simulink library "Navigation_Lib"  (Simulink 7.5)
settings: Solver=ode45  SolverMode=SingleTasking  StartTime=0.0  StopTime=10.0  RelTol=1e-3
values from neighbouring files (symbols this model uses):
  Env =     [UAV_modelconfig.mat]
undefined symbols (not defined in the file or in its folder): Earth, WGS84
libraries: simulink x2, aerolibtransform2 x1
settings Model: Creator=Paul Freeman  LastModifiedBy=ultrastick

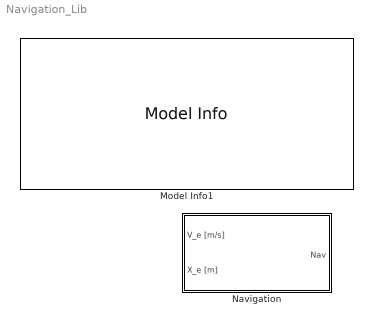
== system Navigation_Lib ==
  Model Info1 : simulink/Model-Wide Utilities/Model Info  SystemSampleTime=-1  InitialBlockCM=None  BlockCM=None  Frame=on  DisplayStringWithTags=|  HorizontalTextAlignment=Left  LeftAlignmentValue=0.02  SourceBlockDiagram=Navigation_Lib  TagMaxNumber=20
      | MODEL INFORMATION
      | Navigation Library
      | 
      | University of Minnesota
      | Aerospace Engineering and Mechanics
      | Copyright 2011 Regents of the University of Minnesota. All rights reserved.
      | 
      | == SVN Info ==
      | %<ModelVersion>
      | Last modified by %<LastModifiedBy> on %<LastModificationDate>
  Navigation : Subsystem  Description=|
      | This model produces the followng navigation data for the UAV flight:
      |                                                                     
      | * Geodetic Latitude                                                 
      | * Geodetic Longitude                                                
      | * Geodetic Altitude                                                 
      | * Altitude above Mean Sea Level                                     
      | * Gravitational acceleration vector

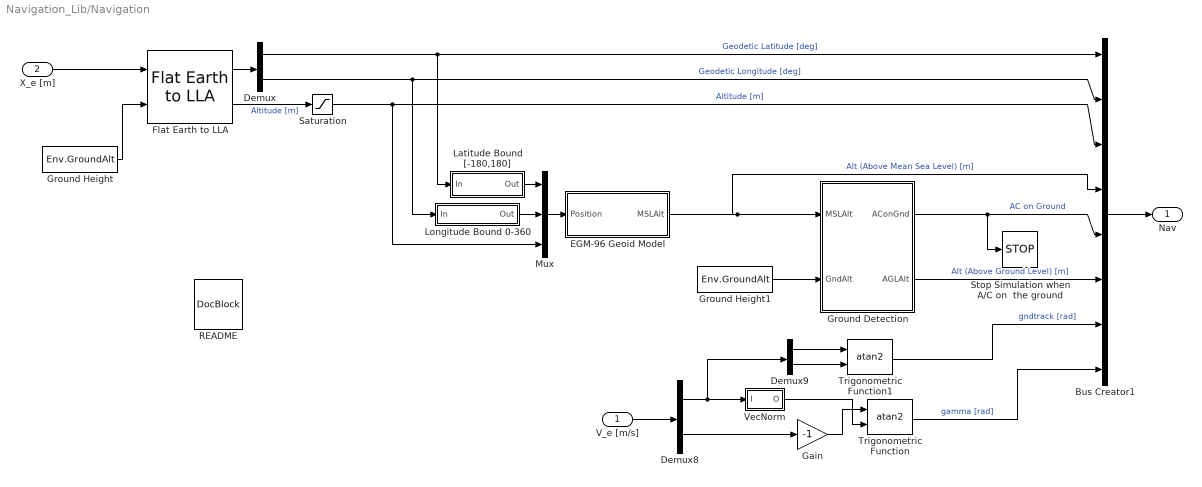
== system Navigation_Lib/Navigation ==
  V_e [m/s] : Inport  OutDataType=sfix(16)  OutScaling=2^0
  X_e [m] : Inport  Port=2  OutDataType=sfix(16)  OutScaling=2^0
  Bus Creator1 : BusCreator  Inputs=8
  Demux : Demux  Outputs=2
  Demux8 : Demux  Outputs=[2 1]
  Demux9 : Demux  Outputs=2
  EGM-96 Geoid Model : Subsystem  mask(EGM-96 geoid undulation model){}
      mask help: Computes the MSL (mean sea level) altitude as a function of position.
      mask init:
      | load('egm96');
      mask Help:
      | The block computes the mean-sea-level altitude relative to the WGS-84 geoid.
      | <P><B>Inputs:</B>
      | <LI>Position = the 3x1 vector of aircraft location [Latitude Longitude Altitude], in [rad rad m]</LI>
      | </P>
      | <P><B>Output:</B>
      | <LI>MSLAlt = the mean-sea-level altitude, in m</LI>
      | </P>
  Flat Earth to LLA : aerolibtransform2/Flat Earth to LLA  SystemSampleTime=-1  units=Metric (MKS)  ptype=Earth (WGS84)  F=1/298.257223563  R=6378137  LL0=TrimCondition.LLIni  psi=0
  Gain : Gain  Gain=-1  ParameterDataType=fixdt(1, 16)  ParameterScaling=2^0  OutDataType=fixdt(1, 16)  OutScaling=2^0
  Ground Detection : Subsystem
      mask Type: Ground detection
      mask Description: Computes altitude above ground and sets a flag if AGL is negative.
      mask Help:
      | The block computes the altitude above ground (AGL) and sets a flag if the AGL is negative (used for ground contact detection).
      | <P><B>Inputs:</B>
      | <LI>MSLAlt = the altitude measured from mean-sea-level, in meters</LI>
      | <LI>GndAlt = the altitude of the terrain (above MSL) at current location, in meters</LI>
      | </P>
      | <P><B>Output:</B>
      | <LI>AConGnd = the aircraft-on-ground flag (0 if aircraft above ground, 1 if aircraft on the ground)</LI>
      | <LI>AGLAlt = the altitude of the aircraft above ground</LI>
      | </P>
  Ground Height : Constant  Value=Env.GroundAlt  OutDataType=sfix(16)  OutScaling=2^0
  Ground Height1 : Constant  Value=Env.GroundAlt  OutDataType=sfix(16)  OutScaling=2^0
  Latitude Bound [-180,180] : Subsystem
  Longitude Bound 0-360 : Subsystem
      mask Type: Longitude bound
      mask Description: Bounds the longitude to [0, 2pi]. When 0 bound is exceeded the longitude wraps back to 2pi; when the 2pi bound is exceeded the longitude wraps back to 0.
  Mux : Mux  Inputs=3
  README : simulink/Model-Wide Utilities/DocBlock  SystemSampleTime=-1  DocumentType=Text
      content=|
      | Navigation
      |
      | This block is library link that contains the navigational model and
      | equations. Included are equations relating the flat Earth position to
      | latitude/longitude, a simplified 2D table lookup version of the EGM-96
      | Geoid model for computation of MSL/AGL altitudes, and computation of
      | flight path and ground track angles.
  Saturation : Saturate  UpperLimit=Inf  LowerLimit=0  OutDataType=fixdt(1, 16)  OutScaling=2^0
  Stop Simulation when A/C on  the ground : Stop
  Trigonometric Function : Trigonometry  Operator=atan2
  Trigonometric Function1 : Trigonometry  Operator=atan2
  VecNorm : Subsystem
  Nav : Outport  OutDataType=sfix(16)  OutScaling=2^0
  wires:
  Flat Earth to LLA/1 -> Demux/1
  Flat Earth to LLA/2 -> Saturation/1  "Altitude [m]"
  Demux/1 -> Bus Creator1/1, Latitude Bound [-180,180]/1(In)  "Geodetic Latitude [deg]"
  Demux/2 -> Bus Creator1/2, Longitude Bound 0-360/1(In)  "Geodetic Longitude [deg]"
  X_e [m]/1 -> Flat Earth to LLA/1
  Ground Height/1 -> Flat Earth to LLA/2
  Bus Creator1/1 -> Nav/1
  EGM-96 Geoid Model/1(MSLAlt) -> Ground Detection/1(MSLAlt), Bus Creator1/4  "Alt (Above Mean Sea Level) [m]"
  Ground Height1/1 -> Ground Detection/2(GndAlt)
  Ground Detection/1(AConGnd) -> Stop Simulation when A/C on  the ground/1, Bus Creator1/5  "AC on Ground"
  Saturation/1 -> Bus Creator1/3, Mux/3  "Altitude [m]"
  Mux/1 -> EGM-96 Geoid Model/1(Position)
  Ground Detection/2(AGLAlt) -> Bus Creator1/6  "Alt (Above Ground Level) [m]"
  V_e [m/s]/1 -> Demux8/1
  Demux8/2 -> Gain/1
  VecNorm/1(O) -> Trigonometric Function/2
  Trigonometric Function/1 -> Bus Creator1/8  "gamma [rad]"
  Demux9/2 -> Trigonometric Function1/2
  Trigonometric Function1/1 -> Bus Creator1/7  "gndtrack [rad]"
  Demux8/1 -> VecNorm/1(I), Demux9/1
  Demux9/1 -> Trigonometric Function1/1
  Longitude Bound 0-360/1(Out) -> Mux/2
  Latitude Bound [-180,180]/1(Out) -> Mux/1
  Gain/1 -> Trigonometric Function/1

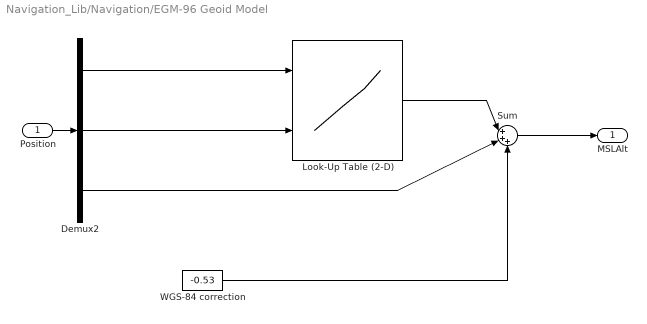
== system Navigation_Lib/Navigation/EGM-96 Geoid Model ==
  Position : Inport  OutDataType=sfix(16)  OutScaling=2^0
  Demux2 : Demux  Outputs=3
  Look-Up Table (2-D) : Lookup2D  RowIndex=Lat  ColumnIndex=Lon  Table=Alterr'  OutDataType=sfix(16)  OutScaling=2^0  SaturateOnIntegerOverflow=on  InputSameDT=on
  Sum : Sum  Inputs=|+++  OutDataType=fixdt(1, 16)  OutScaling=2^0
  WGS-84 correction : Constant  Value=-0.53  OutDataType=sfix(16)  OutScaling=2^0
  MSLAlt : Outport
  wires:
  Demux2/2 -> Look-Up Table (2-D)/2
  Demux2/1 -> Look-Up Table (2-D)/1
  Position/1 -> Demux2/1
  Demux2/3 -> Sum/2
  Sum/1 -> MSLAlt/1
  Look-Up Table (2-D)/1 -> Sum/1
  WGS-84 correction/1 -> Sum/3

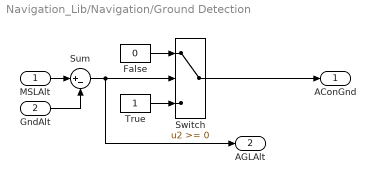
== system Navigation_Lib/Navigation/Ground Detection ==
  MSLAlt : Inport
  GndAlt : Inport  Port=2
  False : Constant  Value=0
  Sum : Sum  Inputs=|+-  SaturateOnIntegerOverflow=on  InputSameDT=on  OutDataTypeStr=Inherit: Same as first input
  Switch : Switch  SaturateOnIntegerOverflow=on  InputSameDT=on
  True : Constant
  AConGnd : Outport
  AGLAlt : Outport  Port=2
  wires:
  Switch/1 -> AConGnd/1
  True/1 -> Switch/3
  False/1 -> Switch/1
  Sum/1 -> AGLAlt/1, Switch/2
  GndAlt/1 -> Sum/2
  MSLAlt/1 -> Sum/1

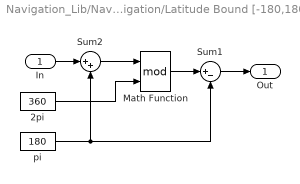
== system Navigation_Lib/Navigation/Latitude Bound [-180,180] ==
  In : Inport  OutDataType=sfix(16)  OutScaling=2^0
  2pi : Constant  Value=360  OutDataType=sfix(16)  OutScaling=2^0
  Math Function : Math  Operator=mod  SaturateOnIntegerOverflow=on
  Sum1 : Sum  Inputs=|+-  OutDataType=sfix(16)  OutScaling=2^0  SaturateOnIntegerOverflow=on  InputSameDT=on  OutDataTypeStr=Inherit: Same as first input
  Sum2 : Sum  Inputs=|++  OutDataType=sfix(16)  OutScaling=2^0  SaturateOnIntegerOverflow=on  InputSameDT=on  OutDataTypeStr=Inherit: Same as first input
  pi : Constant  Value=180  OutDataType=sfix(16)  OutScaling=2^0
  Out : Outport
  wires:
  Sum1/1 -> Out/1
  pi/1 -> Sum1/2, Sum2/2
  Sum2/1 -> Math Function/1
  In/1 -> Sum2/1
  2pi/1 -> Math Function/2
  Math Function/1 -> Sum1/1

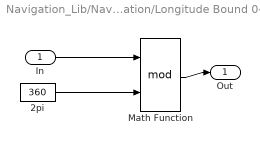
== system Navigation_Lib/Navigation/Longitude Bound 0-360 ==
  In : Inport  OutDataType=sfix(16)  OutScaling=2^0
  2pi : Constant  Value=360  OutDataType=sfix(16)  OutScaling=2^0
  Math Function : Math  Operator=mod  SaturateOnIntegerOverflow=on
  Out : Outport
  wires:
  In/1 -> Math Function/1
  2pi/1 -> Math Function/2
  Math Function/1 -> Out/1

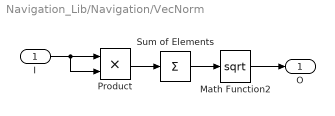
== system Navigation_Lib/Navigation/VecNorm ==
  I : Inport  OutDataType=sfix(16)  OutScaling=2^0
  Math Function2 : Math  Operator=sqrt  OutDataType=sfix(16)  OutScaling=2^0  SaturateOnIntegerOverflow=on
  Product : Product  OutDataType=sfix(16)  OutScaling=2^0  RndMeth=Zero
  Sum of Elements : Sum  Inputs=+  OutDataType=sfix(16)  OutScaling=2^-10
  O : Outport  OutDataType=sfix(16)  OutScaling=2^0
  wires:
  Math Function2/1 -> O/1
  I/1 -> Product/1, Product/2
  Product/1 -> Sum of Elements/1
  Sum of Elements/1 -> Math Function2/1
